simulink model "AdaptiveSync_2_2"  (R2016a)
settings: Solver=ode23tb  SolverMode=SingleTasking  StartTime=0.0  StopTime=10  RelTol=1e-3
values from neighbouring files (symbols this model uses):
  A1 = [0,1;-2,-1]    [Adaptive_Synchronization.m]
  A2 = [0,1;-2.5,-0.75]    [Adaptive_Synchronization.m]
  A3 = [0,1;-2,-1.25]    [Adaptive_Synchronization.m]
  A4 = [0,1;-1,-0.5]    [Adaptive_Synchronization.m]
  A5 = [0,1;-1,-0.75]    [Adaptive_Synchronization.m]
  Aer = kron(L,eye(2))    [Adaptive_Synchronization.m]
  Am = [0 1;-(0.7)^2, 0]    [Adaptive_Synchronization.m]
  B1 = [0;1]    [Adaptive_Synchronization.m]
  B2 = [0;1]    [Adaptive_Synchronization.m]
  B3 = [0;1]    [Adaptive_Synchronization.m]
  B4 = [0;1]    [Adaptive_Synchronization.m]
  B5 = [0;1]    [Adaptive_Synchronization.m]
  Bm = [0;1]    [Adaptive_Synchronization.m]
  Cm = eye(2)    [Adaptive_Synchronization.m]
  Dm = [0;0]    [Adaptive_Synchronization.m]
  F = [-10 -10]    [Adaptive_Synchronization.m]
  k1 = Am(2,:)-A1(2,:)    [Adaptive_Synchronization.m]
  k2 = Am(2,:)-A2(2,:)    [Adaptive_Synchronization.m]
  k3 = Am(2,:)-A3(2,:)    [Adaptive_Synchronization.m]
  k4 = Am(2,:)-A4(2,:)    [Adaptive_Synchronization.m]
  k5 = Am(2,:)-A5(2,:)    [Adaptive_Synchronization.m]
  l1 = 1    [Adaptive_Synchronization.m]
  l2 = 1    [Adaptive_Synchronization.m]
  l3 = 1    [Adaptive_Synchronization.m]
  l4 = 1    [Adaptive_Synchronization.m]
  l5 = 1    [Adaptive_Synchronization.m]
  x01 = [-0.5;1]    [Adaptive_Synchronization.m]
  x02 = [0.5;-1]    [Adaptive_Synchronization.m]
  x03 = [1;0.5]    [Adaptive_Synchronization.m]
  x04 = [-1;-0.5]    [Adaptive_Synchronization.m]
  x05 = [0;0]    [Adaptive_Synchronization.m]
  x0m = [0;1]    [Adaptive_Synchronization.m]
settings Model: Creator=tdvos  LastModifiedBy=danielvos
settings SolverCC: ZeroCrossAlgorithm=Adaptive
settings DebuggingCC: SFUnexpectedBacktrackingDiag=error  SFNoUnconditionalDefaultTransitionDiag=error
settings GRTTargetCC: TargetLangStandard=C99 (ISO)  GeneratePreprocessorConditionals=Use local settings
settings ConfigComp: CovMetricSettings=dwe  CovHtmlReporting=off  CovSaveCumulativeToWorkspaceVar=off  CovSaveSingleToWorkspaceVar=off  CovExternalEMLEnable=on

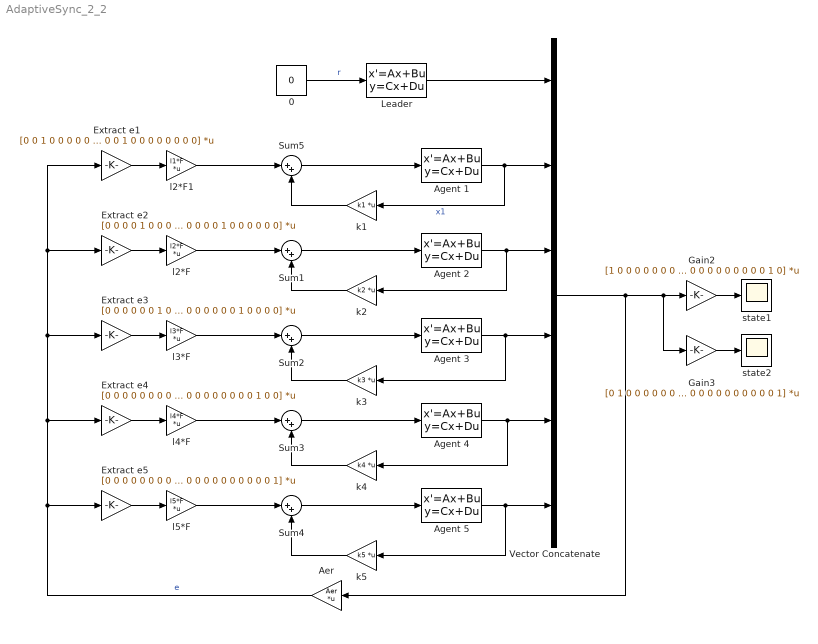
== system AdaptiveSync_2_2 ==
  0 : Constant  Value=0
  Aer : Gain  Gain=Aer  Multiplication=Matrix(K*u)
  Agent 1 : StateSpace  A=A1  B=B1  C=eye(2)  D=zeros(2,1)  X0=x01
  Agent 2 : StateSpace  A=A2  B=B2  C=eye(2)  D=zeros(2,1)  X0=x02
  Agent 3 : StateSpace  A=A3  B=B3  C=eye(2)  D=zeros(2,1)  X0=x03
  Agent 4 : StateSpace  A=A4  B=B4  C=eye(2)  D=zeros(2,1)  X0=x04
  Agent 5 : StateSpace  A=A5  B=B5  C=eye(2)  D=zeros(2,1)  X0=x05
  Extract e1 : Gain  Gain=[0 0 1 0 0 0 0 0 0 0 0 0; 0 0 0 1 0 0 0 0 0 0 0 0]  Multiplication=Matrix(K*u)
  Extract e2 : Gain  Gain=[0 0 0 0 1 0 0 0 0 0 0 0; 0 0 0 0 0 1 0 0 0 0 0 0]  Multiplication=Matrix(K*u)
  Extract e3 : Gain  Gain=[0 0 0 0 0 0 1 0 0 0 0 0; 0 0 0 0 0 0 0 1 0 0 0 0]  Multiplication=Matrix(K*u)
  Extract e4 : Gain  Gain=[0 0 0 0 0 0 0 0 1 0 0 0; 0 0 0 0 0 0 0 0 0 1 0 0]  Multiplication=Matrix(K*u)
  Extract e5 : Gain  Gain=[0 0 0 0 0 0 0 0 0 0 1 0; 0 0 0 0 0 0 0 0 0 0 0 1]  Multiplication=Matrix(K*u)
  Gain2 : Gain  Gain=[1 0 0 0 0 0 0 0 0 0 0 0;0 0 1 0 0 0 0 0 0 0 0 0;0 0 0 0 1 0 0 0 0 0 0 0;0 0 0 0 0 0 1 0 0 0 0 0;0 0 0 0 0 0 0 0 1 0 0 0;0 0 0 0 0 0 0 0 0 0 1 0]  Multiplication=Matrix(K*u)
  Gain3 : Gain  Gain=[0 1 0 0 0 0 0 0 0 0 0 0;0 0 0 1 0 0 0 0 0 0 0 0;0 0 0 0 0 1 0 0 0 0 0 0;0 0 0 0 0 0 0 1 0 0 0 0;0 0 0 0 0 0 0 0 0 1 0 0; 0 0 0 0 0 0 0 0 0 0 0 1]  Multiplication=Matrix(K*u)
  Leader : StateSpace  A=Am  B=Bm  C=Cm  D=Dm  X0=x0m
  Sum{1..5} (5 alike) : Sum  Inputs=|++
  Vector Concatenate : Concatenate  NumInputs=6
  k1 : Gain  Gain=k1  Multiplication=Matrix(K*u)
  k2 : Gain  Gain=k2  Multiplication=Matrix(K*u)
  k3 : Gain  Gain=k3  Multiplication=Matrix(K*u)
  k4 : Gain  Gain=k4  Multiplication=Matrix(K*u)
  k5 : Gain  Gain=k5  Multiplication=Matrix(K*u)
  l2*F : Gain  Gain=l2*F  Multiplication=Matrix(K*u)
  l2*F1 : Gain  Gain=l1*F  Multiplication=Matrix(K*u)
  l3*F : Gain  Gain=l3*F  Multiplication=Matrix(K*u)
  l4*F : Gain  Gain=l4*F  Multiplication=Matrix(K*u)
  l5*F : Gain  Gain=l5*F  Multiplication=Matrix(K*u)
  state1 : Scope
  state2 : Scope
  wires:
  Agent 1/1 -> k1/1, Vector Concatenate/2  "x1"
  Agent 2/1 -> k2/1, Vector Concatenate/3
  Agent 3/1 -> k3/1, Vector Concatenate/4
  Agent 4/1 -> k4/1, Vector Concatenate/5
  Agent 5/1 -> k5/1, Vector Concatenate/6
  Aer/1 -> Extract e1/1, Extract e2/1, Extract e3/1, Extract e4/1, Extract e5/1  "e"
  Extract e2/1 -> l2*F/1
  Extract e3/1 -> l3*F/1
  Extract e4/1 -> l4*F/1
  Extract e5/1 -> l5*F/1
  l2*F/1 -> Sum1/1
  l3*F/1 -> Sum2/1
  l4*F/1 -> Sum3/1
  l5*F/1 -> Sum4/1
  Sum2/1 -> Agent 3/1
  Sum1/1 -> Agent 2/1
  Sum3/1 -> Agent 4/1
  Sum4/1 -> Agent 5/1
  k2/1 -> Sum1/2
  k3/1 -> Sum2/2
  k4/1 -> Sum3/2
  k5/1 -> Sum4/2
  Leader/1 -> Vector Concatenate/1
  k1/1 -> Sum5/2
  Sum5/1 -> Agent 1/1
  Extract e1/1 -> l2*F1/1
  l2*F1/1 -> Sum5/1
  0/1 -> Leader/1  "r"
  Gain3/1 -> state2/1
  Vector Concatenate/1 -> Gain3/1, Gain2/1, Aer/1
  Gain2/1 -> state1/1
